simulink library "TopDownRFReceiverDesignLib"  (R2024a)
settings: Solver=VariableStepAuto  StartTime=0.0  StopTime=10.0  RelTol=1e-3
undefined symbols (not defined in the file or in its folder): bitRate, chipRate, oversampling
libraries: commrandsrc3 x2, commdigbbndpm3 x2, dspmathops x2, simulink_extras x2, simulink x1, dspfdesign x1, commfilt2 x1, dspsigops x1
settings Model: Creator=The MathWorks, Inc.  LastModifiedBy=gzucchel
settings SolverCC: AlgebraicLoopSolver=TrustRegion
settings OptimizationCC: ReuseModelBlockBuffer=off
settings DebuggingCC: UnconnectedInputMsg=warning  UnconnectedOutputMsg=warning  UnconnectedLineMsg=warning  SymbolicDimsDataTypeCodeGenerationDiagnostic=none
settings ModelReferenceCC: EnableRefExpFcnMdlSchedulingChecks=on
settings RTWCC: GPUComputeCapability=3.5  DLArmComputeVersion=19.05

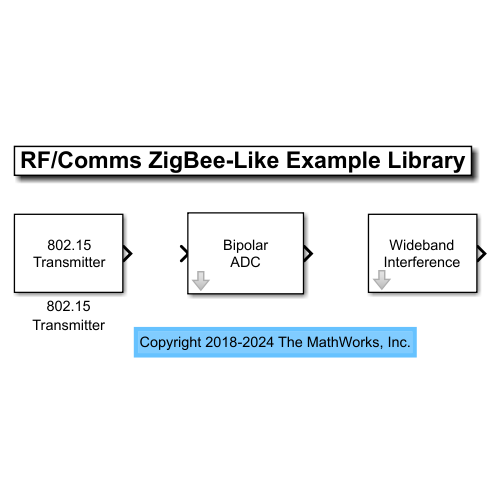
[thumbnail: Simulink's stored preview of the top-level diagram]
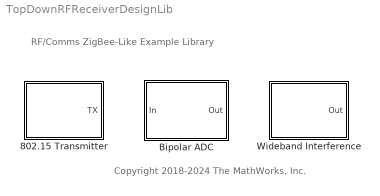
== system TopDownRFReceiverDesignLib ==
  note: RF/Comms ZigBee-Like Example Library
  note: Copyright 2018-2024 The MathWorks, Inc.
  802.15 Transmitter : Subsystem
      mask Display: disp('802.15\nTransmitter')
  Bipolar ADC : Subsystem  mask(Analog-to-Digital Converter){FS_V=sqrt(10^((0-30)/10)), N=10}
      mask prompts: FS_V "Full scale voltage (FSV):"; N "Number of bits (N):"
      mask help: Quantize the input signal with a bipolar ADC. The output levels are floating point numbers in the set of -FSV:LSB:FSV-LSB, where LSB=FSV/2^(N-1) and N is the number of bits. This block is useful to simulate quantization and saturation effects of an ADC on the input signal.
      mask init:
      | LSB=FS_V/(2^(N-1));
      | MAX=FS_V-LSB;
      | MIN=-FS_V;
      settings: LibrarySourceBlock=commdemoslib/Bipolar ADC
      mask Display: disp('Bipolar\nADC')
  Wideband Interference : Subsystem  mask{Pout=-30}
      mask prompts: Pout "Output power (dBm)"
      mask Display: disp('Wideband\nInterference')

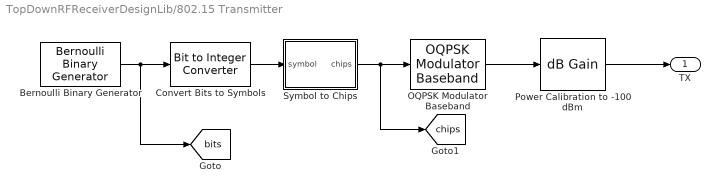
== system TopDownRFReceiverDesignLib/802.15 Transmitter ==
  Bernoulli Binary Generator : commrandsrc3/Bernoulli Binary Generator  ProbabilityOfZero=0.5  SeedSource=Parameter  Seed=73  SampleTime=1/bitRate  SamplesPerFrame=spf  OutputDataType=double  SimulateUsing=Interpreted execution
  Convert Bits to Symbols : simulink/Logic and Bit Operations/Bit to Integer Converter  nbits=4  bitOrder=MSB first  signedOutputValues=Unsigned  outDtype=Inherit via internal rule  outDtypeSigned=Inherit via internal rule
      settings: LibrarySourceBlock=|
      | commutil2/Bit to Integer
      | Converter
  OQPSK Modulator Baseband : commdigbbndpm3/OQPSK Modulator Baseband  InType=Bit  Ph=0  Mapping=Gray  pulseShape=Half sine  num=[0.7071, 0.7071]  rolloff=0.2  filterSpan=10  sps=sps  RateOptions=Enforce single-rate processing  outDtype=double
  Power Calibration to -100 dBm : dspmathops/dB Gain  dB="-130  % power of preceding block is 1 W"  intype=Amplitude
  Symbol to Chips : MATLAB Function  TreatAsAtomicUnit=on
  TX : Outport  VectorParamsAs1DForOutWhenUnconnected=off
  tag scope: bits=global, chips=global
  wires:
  Power Calibration to -100 dBm/1 -> TX/1
  OQPSK Modulator Baseband/1 -> Power Calibration to -100 dBm/1
  Convert Bits to Symbols/1 -> Symbol to Chips/1(symbol)
  Symbol to Chips/1(chips) -> OQPSK Modulator Baseband/1, [chips]
  Bernoulli Binary Generator/1 -> Convert Bits to Symbols/1, [bits]

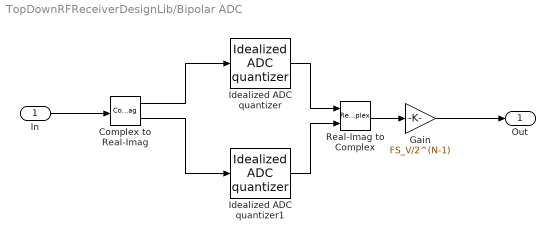
== system TopDownRFReceiverDesignLib/Bipolar ADC ==
  In : Inport
  Complex to Real-Imag : ComplexToRealImag
  Gain : Gain  Gain=FS_V/2^(N-1)
  Idealized ADC quantizer : simulink_extras/Additional Discrete/Idealized ADC quantizer  NumberOfConverterBits=N  Vmin=-FS_V  Vmax=FS_V  OutputDataType=double  OutputNegativeValues=on
  Idealized ADC quantizer1 : simulink_extras/Additional Discrete/Idealized ADC quantizer  NumberOfConverterBits=N  Vmin=-FS_V  Vmax=FS_V  OutputDataType=double  OutputNegativeValues=on
  Real-Imag to Complex : RealImagToComplex
  Out : Outport  VectorParamsAs1DForOutWhenUnconnected=off
  wires:
  In/1 -> Complex to Real-Imag/1
  Real-Imag to Complex/1 -> Gain/1
  Complex to Real-Imag/1 -> Idealized ADC quantizer/1
  Idealized ADC quantizer/1 -> Real-Imag to Complex/1
  Complex to Real-Imag/2 -> Idealized ADC quantizer1/1
  Idealized ADC quantizer1/1 -> Real-Imag to Complex/2
  Gain/1 -> Out/1

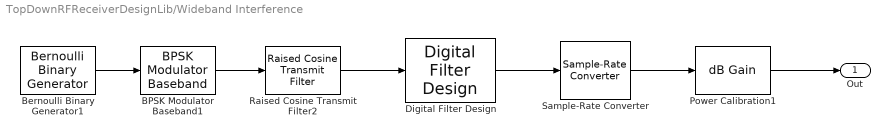
== system TopDownRFReceiverDesignLib/Wideband Interference ==
  BPSK Modulator Baseband1 : commdigbbndpm3/BPSK Modulator Baseband  Ph=0  outDtype=double  outWordLen=16  outUDDataType=sfix(16)  outFracLenMode=Best precision  outFracLen=15  outDataTypeStr=double  outLastDataTypeStr=double
  Bernoulli Binary Generator1 : commrandsrc3/Bernoulli Binary Generator  ProbabilityOfZero=0.5  SeedSource=Parameter  Seed=612  SampleTime="1/4e6  % 1/3.846e6"  SamplesPerFrame="640  % 1923"  OutputDataType=double  SimulateUsing=Interpreted execution
  Digital Filter Design : dspfdesign/Digital Filter Design  mwdsp_browser_bugfix_var=off
  Power Calibration1 : dspmathops/dB Gain  dB=10.2-30+Pout  intype=Amplitude
  Raised Cosine Transmit Filter2 : commfilt2/Raised Cosine Transmit Filter  filtType=Square root  R=0.2  filtSpan=10  N=10  filterGain=1  InputProcessing=Columns as channels (frame based)  RateOptions=Allow multirate processing  framing=Mute  checkCoeff=off  variableName=rcTxFilt2  checkGain=Normalized  sampMode=Mute  saveAsFlag=0  currentFiltSpan=10  D=(10)/2  launchFVT=on  roundingMode=Floor  overflowMode=off  coeffDataTypeStr=Inherit: Same word length as input  coeffMin=[]  coeffMax=[]  coeffLastDataTypeStr=Inherit: Same word length as input  outputDataTypeStr=Inherit: Same as accumulator  outputMin=[]  outputMax=[]  outputLastDataTypeStr=Inherit: Same as accumulator
  Sample-Rate Converter : dspsigops/Sample-Rate Converter  InputSampleRate="40e6  % 38.46e6"  OutputSampleRate=2*chipRate*oversampling  OutputRateTolerance=0  Bandwidth="2*4  % 2*3.846"  StopbandAttenuation=60  AllowArbitraryInputLength=off  SimulateUsing=Code generation
  Out : Outport  VectorParamsAs1DForOutWhenUnconnected=off
  wires:
  Power Calibration1/1 -> Out/1
  Sample-Rate Converter/1 -> Power Calibration1/1
  Raised Cosine Transmit Filter2/1 -> Digital Filter Design/1
  Bernoulli Binary Generator1/1 -> BPSK Modulator Baseband1/1
  BPSK Modulator Baseband1/1 -> Raised Cosine Transmit Filter2/1
  Digital Filter Design/1 -> Sample-Rate Converter/1

== matlab function TopDownRFReceiverDesignLib/802.15 Transmitter/Symbol to Chips ==
  data: symbol input; chips output size=[32 1]
function chips = sym2chips(symbol)
  chipMap = ...
     [1 1 0 1 1 0 0 1 1 1 0 0 0 0 1 1 0 1 0 1 0 0 1 0 0 0 1 0 1 1 1 0;
      1 1 1 0 1 1 0 1 1 0 0 1 1 1 0 0 0 0 1 1 0 1 0 1 0 0 1 0 0 0 1 0;
      0 0 1 0 1 1 1 0 1 1 0 1 1 0 0 1 1 1 0 0 0 0 1 1 0 1 0 1 0 0 1 0;
      0 0 1 0 0 0 1 0 1 1 1 0 1 1 0 1 1 0 0 1 1 1 0 0 0 0 1 1 0 1 0 1;
      0 1 0 1 0 0 1 0 0 0 1 0 1 1 1 0 1 1 0 1 1 0 0 1 1 1 0 0 0 0 1 1;
      0 0 1 1 0 1 0 1 0 0 1 0 0 0 1 0 1 1 1 0 1 1 0 1 1 0 0 1 1 1 0 0;
      1 1 0 0 0 0 1 1 0 1 0 1 0 0 1 0 0 0 1 0 1 1 1 0 1 1 0 1 1 0 0 1;
      1 0 0 1 1 1 0 0 0 0 1 1 0 1 0 1 0 0 1 0 0 0 1 0 1 1 1 0 1 1 0 1;
      1 0 0 0 1 1 0 0 1 0 0 1 0 1 1 0 0 0 0 0 0 1 1 1 0 1 1 1 1 0 1 1;
      1 0 1 1 1 0 0 0 1 1 0 0 1 0 0 1 0 1 1 0 0 0 0 0 0 1 1 1 0 1 1 1;
      0 1 1 1 1 0 1 1 1 0 0 0 1 1 0 0 1 0 0 1 0 1 1 0 0 0 0 0 0 1 1 1;
      0 1 1 1 0 1 1 1 1 0 1 1 1 0 0 0 1 1 0 0 1 0 0 1 0 1 1 0 0 0 0 0;
      0 0 0 0 0 1 1 1 0 1 1 1 1 0 1 1 1 0 0 0 1 1 0 0 1 0 0 1 0 1 1 0;
      0 1 1 0 0 0 0 0 0 1 1 1 0 1 1 1 1 0 1 1 1 0 0 0 1 1 0 0 1 0 0 1;
      1 0 0 1 0 1 1 0 0 0 0 0 0 1 1 1 0 1 1 1 1 0 1 1 1 0 0 0 1 1 0 0;
      1 1 0 0 1 0 0 1 0 1 1 0 0 0 0 0 0 1 1 1 0 1 1 1 1 0 1 1 1 0 0 0];

 chips = chipMap(1+symbol,:)'; % +1 for 1-based indexing
